simulink model "sum_1"  (R2016b)
settings: Solver=VariableStepAuto  StartTime=0.0  StopTime=10.0  RelTol=1e-3
libraries: xbsIndex_r4 x39, simulink x1, dspswit3 x1
settings Model: Creator=root  LastModifiedBy=root

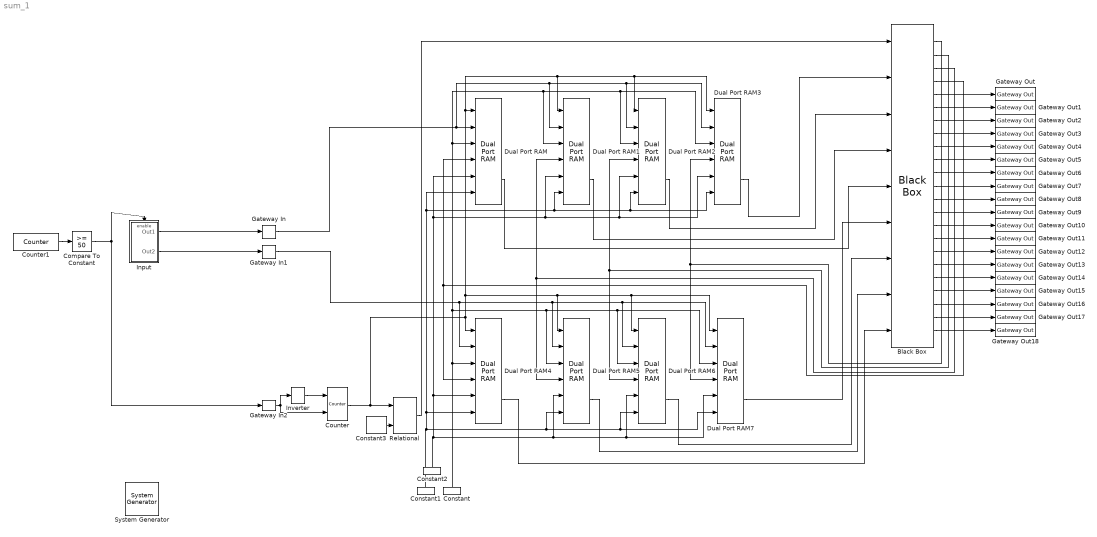
== system sum_1 ==
  " System Generator" : xbsIndex_r4/ System Generator  Tag=genX  xilinxfamily=virtex7  part=xc7vx485t  speed=-2  package=ffg1761  synthesis_tool=Vivado  clock_wrapper=Clock Enables  directory=./netlist  proj_type=Vivado  Synth_file=Vivado Synthesis Defaults  Impl_file=Vivado Implementation Defaults  testbench=off  simulink_period=1/(70e6)  sysclk_period=1000/70  dcm_input_clock_period=10  incr_netlist=off  trim_vbits=Everywhere in SubSystem  dbl_ovrd=According to Block Masks  core_generation=According to Block Masks  run_coregen=off  deprecated_control=off  eval_field=0  block_type=sysgen
  Black Box : xbsIndex_r4/Black Box  init_code=stage3_config  sim_method=ISE Simulator  verbose=off  block_type=blackbox2
  Compare To Constant : simulink/Logic and Bit Operations/Compare To Constant  relop=>=  const=50  OutDataTypeStr=boolean
  Constant : xbsIndex_r4/Constant  const=1  gui_display_data_type=Boolean  arith_type=Boolean  n_bits=16  bin_pt=14  preci_type=Single  exp_width=8  frac_width=24  explicit_period=off  period=1  equ=P=C  opselect=C  inp2=PCIN>>17  opr=+  inp1=P  carry=CIN  dbl_ovrd=off  block_type=constant
  Constant1 : xbsIndex_r4/Constant  const=0  gui_display_data_type=Boolean  arith_type=Boolean  n_bits=16  bin_pt=14  preci_type=Single  exp_width=8  frac_width=24  explicit_period=off  period=1  equ=P=C  opselect=C  inp2=PCIN>>17  opr=+  inp1=P  carry=CIN  dbl_ovrd=off  block_type=constant
  Constant2 : xbsIndex_r4/Constant  const=0  gui_display_data_type=Fixed-point  arith_type=Signed (2's comp)  n_bits=12  bin_pt=0  preci_type=Single  exp_width=8  frac_width=24  explicit_period=off  period=1  equ=P=C  opselect=C  inp2=PCIN>>17  opr=+  inp1=P  carry=CIN  dbl_ovrd=off  block_type=constant
  Constant3 : xbsIndex_r4/Constant  const=1999  gui_display_data_type=Fixed-point  arith_type=Signed (2's comp)  n_bits=16  bin_pt=0  preci_type=Single  exp_width=8  frac_width=24  explicit_period=on  period=1/(70e6)  equ=P=C  opselect=C  inp2=PCIN>>17  opr=+  inp1=P  carry=CIN  dbl_ovrd=off  block_type=constant
  Counter : xbsIndex_r4/Counter  cnt_type=Free Running  cnt_to=Inf  operation=Up  start_count=0  cnt_by_val=1  arith_type=Unsigned  n_bits=16  bin_pt=0  load_pin=off  rst=on  en=on  explicit_period=off  period=1  use_behavioral_HDL=off  implementation=Fabric  dbl_ovrd=off  block_type=counter
  Counter1 : dspswit3/Counter  Direction=Up  CountEvent=Free running  CounterSize=32 bits  MaxCount=255  InitialCount=0  Output=Count  HitValue=32  ResetInput=off  SamplesPerFrame=1  Ts=1/(2e6)  CntDtype=double  HitDtype=Logical
  Dual Port RAM{,1..7} (8 alike) : xbsIndex_r4/Dual Port RAM  depth=65536  initVector=0  distributed_mem=Block RAM  init_a=0  init_b=0  rst_a=off  rst_b=off  en_a=off  en_b=off  latency=1  write_mode_A=Read After Write  write_mode_B=Read After Write  optimize=Area  dbl_ovrd=off  block_type=dpram
  Gateway In : xbsIndex_r4/Gateway In  gui_display_data_type=Fixed-point  arith_type="Signed  (2's comp)"  n_bits=12  bin_pt=0  preci_type=Single  exp_width=8  frac_width=24  rows=1  columns=1  quantization="Round  (unbiased: +/- Inf)"  overflow=Saturate  period=1/(70e6)  UseAsADC=off  ADCChannel='1'  interface=None  automatic_assignment=on  address_offset=hex2dec('00')  intf_name=''  intf_description=''  default_value=0  timing_constraint=None  locs_specified=off  LOCs={}  io_standard={}  inherit_from_input=off  hdl_port=on  dbl_ovrd=off  block_type=gatewayin
  Gateway In1 : xbsIndex_r4/Gateway In  gui_display_data_type=Fixed-point  arith_type="Signed  (2's comp)"  n_bits=12  bin_pt=0  preci_type=Single  exp_width=8  frac_width=24  rows=1  columns=1  quantization="Round  (unbiased: +/- Inf)"  overflow=Saturate  period=1/(70e6)  UseAsADC=off  ADCChannel='1'  interface=None  automatic_assignment=on  address_offset=hex2dec('00')  intf_name=''  intf_description=''  default_value=0  timing_constraint=None  locs_specified=off  LOCs={}  io_standard={}  inherit_from_input=off  hdl_port=on  dbl_ovrd=off  block_type=gatewayin
  Gateway In2 : xbsIndex_r4/Gateway In  gui_display_data_type=Boolean  arith_type=Boolean  n_bits=12  bin_pt=0  preci_type=Single  exp_width=8  frac_width=24  rows=1  columns=1  quantization="Round  (unbiased: +/- Inf)"  overflow=Saturate  period=1/(2e6)  UseAsADC=off  ADCChannel='1'  interface=None  automatic_assignment=on  address_offset=hex2dec('00')  intf_name=''  intf_description=''  default_value=0  timing_constraint=None  locs_specified=off  LOCs={}  io_standard={}  inherit_from_input=off  hdl_port=on  dbl_ovrd=off  block_type=gatewayin
  Gateway Out{,1..18} (19 alike) : xbsIndex_r4/Gateway Out  inherit_from_input=off  hdl_port=on  rows=1  columns=1  UseAsDAC=off  DACChannel='1'  interface=None  automatic_assignment=on  address_offset=hex2dec('00')  intf_name=''  intf_description=''  timing_constraint=None  locs_specified=off  LOCs={}  io_standard={}  block_type=gatewayout
  "Input " : Subsystem
  Inverter : xbsIndex_r4/Inverter  en=off  latency=0  dbl_ovrd=off  block_type=inv
  Relational : xbsIndex_r4/Relational  mode=a<=b  op_type=Bool  en=off  latency=0  dbl_ovrd=off  block_type=relational
  wires:
  "Input "/1(Out1) -> Gateway In/1
  "Input "/2(Out2) -> Gateway In1/1
  Counter1/1 -> Compare To Constant/1
  Compare To Constant/1 -> Gateway In2/1, "Input "/Enable
  Gateway In2/1 -> Inverter/1, Counter/2
  Gateway In/1 -> Dual Port RAM/2, Dual Port RAM1/2, Dual Port RAM2/2, Dual Port RAM3/2
  Constant/1 -> Dual Port RAM1/3, Dual Port RAM2/3, Dual Port RAM3/3, Dual Port RAM/3, Dual Port RAM5/3, Dual Port RAM6/3, Dual Port RAM7/3, Dual Port RAM4/3
  Black Box/1 -> Dual Port RAM3/4, Dual Port RAM7/4
  Counter/1 -> Relational/1, Dual Port RAM1/1, Dual Port RAM2/1, Dual Port RAM3/1, Dual Port RAM/1, Dual Port RAM5/1, Dual Port RAM7/1, Dual Port RAM6/1, Dual Port RAM4/1
  Constant2/1 -> Dual Port RAM5/5, Dual Port RAM6/5, Dual Port RAM7/5, Dual Port RAM4/5, Dual Port RAM3/5, Dual Port RAM2/5, Dual Port RAM1/5, Dual Port RAM/5
  Constant1/1 -> Dual Port RAM5/6, Dual Port RAM6/6, Dual Port RAM7/6, Dual Port RAM4/6, Dual Port RAM/6, Dual Port RAM1/6, Dual Port RAM2/6, Dual Port RAM3/6
  Gateway In1/1 -> Dual Port RAM4/2, Dual Port RAM5/2, Dual Port RAM7/2, Dual Port RAM6/2
  Black Box/4 -> Dual Port RAM/4, Dual Port RAM4/4
  Black Box/3 -> Dual Port RAM1/4, Dual Port RAM5/4
  Black Box/2 -> Dual Port RAM2/4, Dual Port RAM6/4
  Dual Port RAM3/2 -> Black Box/2
  Dual Port RAM2/2 -> Black Box/3
  Dual Port RAM1/2 -> Black Box/4
  Dual Port RAM/2 -> Black Box/5
  Dual Port RAM7/2 -> Black Box/6
  Dual Port RAM6/2 -> Black Box/7
  Dual Port RAM5/2 -> Black Box/8
  Dual Port RAM4/2 -> Black Box/9
  Inverter/1 -> Counter/1
  Constant3/1 -> Relational/2
  Relational/1 -> Black Box/1
  Black Box/5 -> Gateway Out/1
  Black Box/6 -> Gateway Out1/1
  Black Box/7 -> Gateway Out2/1
  Black Box/8 -> Gateway Out3/1
  Black Box/9 -> Gateway Out4/1
  Black Box/10 -> Gateway Out5/1
  Black Box/11 -> Gateway Out6/1
  Black Box/12 -> Gateway Out7/1
  Black Box/13 -> Gateway Out8/1
  Black Box/14 -> Gateway Out9/1
  Black Box/15 -> Gateway Out10/1
  Black Box/16 -> Gateway Out11/1
  Black Box/17 -> Gateway Out12/1
  Black Box/18 -> Gateway Out13/1
  Black Box/19 -> Gateway Out14/1
  Black Box/20 -> Gateway Out15/1
  Black Box/21 -> Gateway Out16/1
  Black Box/22 -> Gateway Out17/1
  Black Box/23 -> Gateway Out18/1

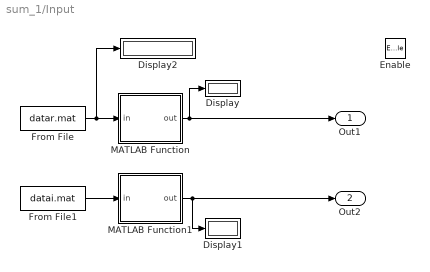
== system sum_1/Input  ==
  Enable : EnablePort
  Display : Display
  Display1 : Display
  Display2 : Display
  From File : FromFile  FileName=datar.mat  SampleTime=1/(2e6)
  From File1 : FromFile  FileName=datai.mat  SampleTime=1/(2e6)
  MATLAB Function : MATLAB Function  TreatAsAtomicUnit=on
  MATLAB Function1 : MATLAB Function  TreatAsAtomicUnit=on
  Out1 : Outport
  Out2 : Outport  Port=2
  wires:
  From File1/1 -> MATLAB Function1/1(in)
  MATLAB Function/1(out) -> Out1/1, Display/1
  From File/1 -> Display2/1, MATLAB Function/1(in)
  MATLAB Function1/1(out) -> Out2/1, Display1/1

== matlab function sum_1/Input /MATLAB Function1 ==
  data: in input; out output
function out=toint(in)
in=in*2^16;
in=round(in);
out=fix(in);

== matlab function sum_1/Input /MATLAB Function ==
  data: in input; out output
function out=toint(in)
in=in*2^16;
in=round(in);
out=fix(in);
